simulink model "SOC_Estimation_vk"  (R2018b)
settings: Solver=ode4  StartTime=0.0  StopTime=5000  FixedStep=1e-3  RelTol=1e-3
libraries: nesl_utility x8, fl_lib x7, ee_lib x2
settings Model: Creator=Suresh  LastModifiedBy=Suresh
settings DataIOCC: ReturnWorkspaceOutputs=on

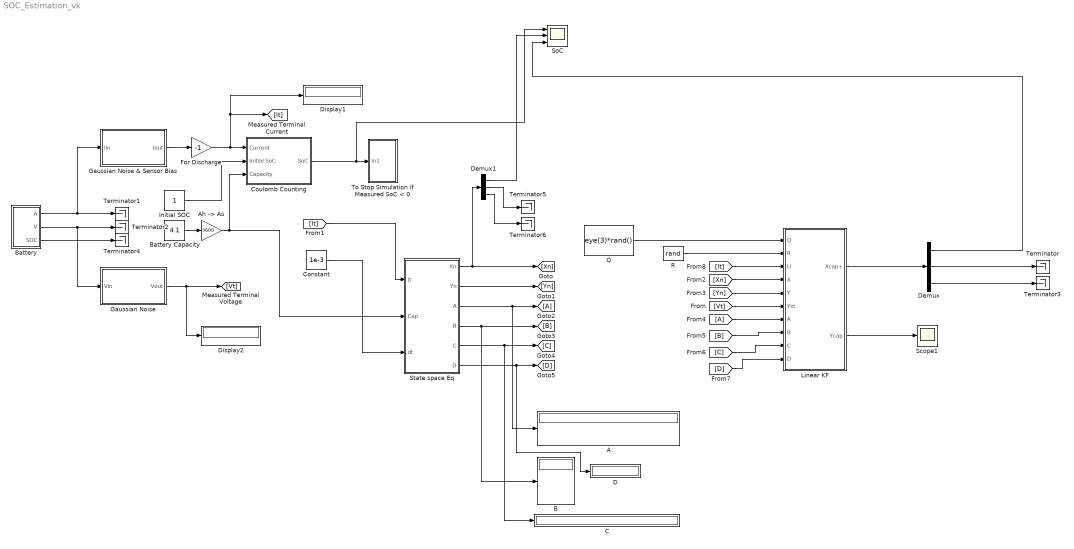
== system SOC_Estimation_vk ==
  A : Display
  "Ah -> As" : Gain  Gain=3600
  B : Display
  Battery : Subsystem
  Battery Capacity : Constant  Value=4.1
  C : Display
  Constant : Constant  Value=1e-3
  "Coulomb Counting " : Subsystem
  D : Display
  Demux : Demux  Outputs=3
  Demux1 : Demux  Outputs=3
  Display1 : Display
  Display2 : Display
  For Discharge : Gain  Gain=-1
  Gaussian Noise : Subsystem
  Gaussian Noise & Sensor Bias : Subsystem
  Initial SOC : Constant
  Linear KF : Subsystem
  Q : Constant  Value=eye(3)*rand()
  R : Constant  Value=rand
  Scope1 : Scope
  SoC : Scope  NumInputPorts=3
  State space Eq : Subsystem
  Terminator{,1..6} (7 alike) : Terminator
  To Stop Simulation if Measured SoC < 0 : Subsystem
  wires:
  Battery/2(V) -> Gaussian Noise/1(Vin), Terminator2/1
  Battery/1(A) -> Gaussian Noise & Sensor Bias/1(Iin), Terminator1/1
  Gaussian Noise & Sensor Bias/1(Iout) -> For Discharge/1
  "Coulomb Counting "/1("SoC ") -> SoC/1, To Stop Simulation if Measured SoC < 0/1(In1)
  Initial SOC/1 -> "Coulomb Counting "/2(Initial SoC)
  Battery/3(SOC) -> Terminator4/1
  Gaussian Noise/1(Vout) -> Display2/1, [Vt]
  Battery Capacity/1 -> "Ah -> As"/1
  For Discharge/1 -> [It], Display1/1, "Coulomb Counting "/1(Current)
  "Ah -> As"/1 -> State space Eq/2(Cap), "Coulomb Counting "/3(Capacity)
  [It] -> State space Eq/1(It)
  Constant/1 -> State space Eq/3(dt)
  State space Eq/1(Xn) -> Demux1/1, [Xn]
  State space Eq/2(Yn) -> [Yn]
  State space Eq/3(A) -> [A], A/1
  State space Eq/4(B) -> [B], B/1
  State space Eq/5(C) -> [C], C/1
  State space Eq/6(D) -> D/1, [D]
  Demux/2 -> Terminator/1
  Demux/3 -> Terminator3/1
  Demux/1 -> SoC/3
  Demux1/1 -> SoC/2
  Demux1/2 -> Terminator5/1
  Demux1/3 -> Terminator6/1
  Q/1 -> Linear KF/1(Q)
  R/1 -> Linear KF/2(R)
  [It] -> Linear KF/3(U)
  [Xn] -> Linear KF/4(X)
  [Yn] -> Linear KF/5(Y)
  [Vt] -> Linear KF/6(Ym)
  [A] -> Linear KF/7(A)
  [B] -> Linear KF/8(B)
  [C] -> Linear KF/9(C)
  [D] -> Linear KF/10(D)
  Linear KF/1(Xcap+) -> Demux/1
  Linear KF/2(Ycap) -> Scope1/1

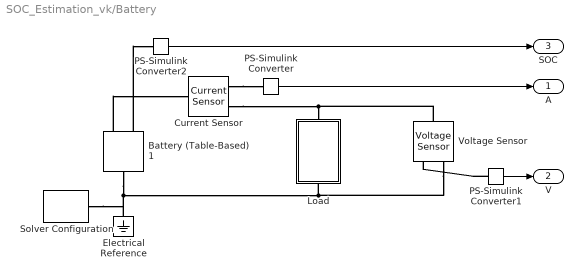
== system SOC_Estimation_vk/Battery ==
  Battery (Table-Based)1 : ee_lib/Sources/Battery (Table-Based)  SOC_vec=[0, .25, .75, 1]  T_vec=[273.15, 298.15, 323.15] K  V0_mat=[3.2, 3.1, 3.14; 3.25, 3.27, 3.3; 3.28, 3.31, 3.34; 3.33, 3.5, 3.59] V  R0_mat=[.03, .015, .002; .04, .017, .008; .039, .012, .006; .027, .013, .021] Ohm  AH_vec=[2.9, 4.1, 4.2] hr*A  prm_leak=1  Rleak_vec=[8000, 7000, 6000] Ohm  prm_dyn=3  R1_mat=[.089, .076, .01; .042, .022, .099; .019, .007, .002; .051, .043, .029] Ohm  tau1_mat=[44, 148, 235; 93, 110, 1000; 19, 27, 133; .5, 22, 3] s  R2_mat=[.014, .382, .407; .028, .006, .007; .014, .007, .006; .333, .956, .912] Ohm  tau2_mat=[1, 44, 5644; 11, 24, 506; 2, 14, 330; 3310, 13419, 30216] s  R3_mat=[.014, .382, .407; .028, .006, .007; .014, .007, .006; .333, .956, .912] Ohm  tau3_mat=[1, 44, 5644; 11, 24, 506; 2, 14, 330; 3310, 13419, 30216] s  R4_mat=[.014, .382, .407; .028, .006, .007; .014, .007, .006; .333, .956, .912] Ohm  tau4_mat=[1, 44, 5644; 11, 24, 506; 2, 14, 330; 3310, 13419, 30216] s  R5_mat=[.014, .382, .407; .028, .006, .007; .014, .007, .006; .333, .956, .912] Ohm  tau5_mat=[1, 44, 5644; 11, 24, 506; 2, 14, 330; 3310, 13419, 30216] s  N0=100  dV0=0  dR0=0  dAH=0  dRleak=0  dR1=0  dR2=0  dR3=0  dR4=0  dR5=0  temperature=298.15 K  i_specify=off  i_priority=None  i=0 A  i_nominal_specify=off  i_nominal_unit=A  i_nominal_value=1  v_specify=off  v_priority=None  v=0 V  v_nominal_specify=off  v_nominal_unit=V  v_nominal_value=1  stateOfCharge_specify=off  stateOfCharge_priority=High  stateOfCharge=1  stateOfCharge_nominal_specify=off  stateOfCharge_nominal_unit=1  stateOfCharge_nominal_value=1  num_cycles_specify=off  num_cycles_priority=High  num_cycles=0  num_cycles_nominal_specify=off  num_cycles_nominal_unit=1  num_cycles_nominal_value=1  thermal_mass=30000 J/K  temperature_specify=off  temperature_priority=High  temperature_nominal_specify=off  temperature_nominal_unit=K  temperature_nominal_value=1
      settings: SourceProductName=Simscape Electrical  SourceProductBaseCode=PS  LogSimulationData=on
  Current Sensor : fl_lib/Electrical/Electrical Sensors/Current Sensor
  Electrical Reference : fl_lib/Electrical/Electrical Elements/Electrical Reference
  Load : Subsystem
  PS-Simulink Converter : nesl_utility/PS-Simulink Converter  PhysicalDomain=network_engine_domain  SubClassName=ps_output  LeftPortType=input  RightPortType=output  PseudoPeriodic=off  Frequencies=[]  Unit=1  AffineConversion=off
  PS-Simulink Converter1 : nesl_utility/PS-Simulink Converter  PhysicalDomain=network_engine_domain  SubClassName=ps_output  LeftPortType=input  RightPortType=output  PseudoPeriodic=off  Frequencies=[]  Unit=1  AffineConversion=off
  PS-Simulink Converter2 : nesl_utility/PS-Simulink Converter  PhysicalDomain=network_engine_domain  SubClassName=ps_output  LeftPortType=input  RightPortType=output  PseudoPeriodic=off  Frequencies=[]  Unit=1  AffineConversion=off
  Solver Configuration : nesl_utility/Solver Configuration  PhysicalDomain=network_engine_domain  SubClassName=solver  LeftPortType=input  RightPortType=generic  Tones=[]  Harmonics=[]  SimulateNoise=off  Profile=off  UseLocalSampling=off  EnableSwitchedLinearOptims=on  FrequencyDomain=off  UseCCode=off  RelTol=0.001  AbsTol=1e-06  MinStep=1e-09  ToWorkspace=off  RevertToSquareIcSolve=off  NumHomotopyIterations=100  PhasorMode=off  PhasorModeNumHarmonics=1  DoDC=off  ResidualTolerance=1e-09  UseLocalSolver=off  LocalSolverChoice=NE_BACKWARD_EULER_ADVANCER  LocalSolverSampleTime=0.001  DoFixedCost=off  MaxNonlinIter=3  MaxModeIter=2  LinearAlgebra=auto  EquationFormulation=NE_TIME_EF  DelaysMemoryBudget=1024  AutomaticFiltering=on  FilteringTimeConstant=0.001  PartitionStorageMethod=AS_NEEDED  PartitionMemoryBudget=1024  PartitionMethod=ROBUST
  Voltage Sensor : fl_lib/Electrical/Electrical Sensors/Voltage Sensor
  A : Outport
  V : Outport  Port=2
  SOC : Outport  Port=3
  wires:
  PS-Simulink Converter/1 -> A/1
  PS-Simulink Converter1/1 -> V/1
  PS-Simulink Converter2/1 -> SOC/1
  connections:
  PS-Simulink Converter1/LConn1 -- Voltage Sensor/RConn1
  Current Sensor/RConn2 -- Voltage Sensor/LConn1 -- Load/LConn1
  Battery (Table-Based)1/LConn1 -- Current Sensor/LConn1
  Current Sensor/RConn1 -- PS-Simulink Converter/LConn1
  Battery (Table-Based)1/LConn2 -- PS-Simulink Converter2/LConn1
  Voltage Sensor/RConn2 -- Load/RConn1 -- Battery (Table-Based)1/RConn1 -- Solver Configuration/RConn1 -- Electrical Reference/LConn1

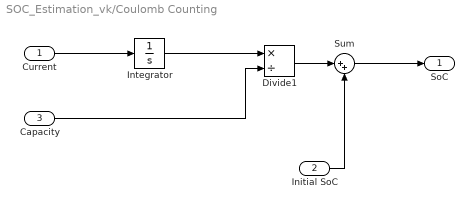
== system SOC_Estimation_vk/Coulomb Counting  ==
  Current : Inport
  Initial SoC : Inport  Port=2
  Capacity : Inport  Port=3
  Divide1 : Product  Inputs=*/
  Integrator : Integrator  LimitOutput=on
  Sum : Sum  Inputs=|++
  "SoC " : Outport
  wires:
  Current/1 -> Integrator/1
  Integrator/1 -> Divide1/1
  Divide1/1 -> Sum/1
  Sum/1 -> "SoC "/1
  Initial SoC/1 -> Sum/2
  Capacity/1 -> Divide1/2

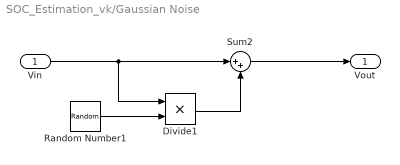
== system SOC_Estimation_vk/Gaussian Noise ==
  Vin : Inport
  Divide1 : Product
  Random Number1 : RandomNumber  Variance=0.000025  Seed=100  SampleTime=1
  Sum2 : Sum  Inputs=|++
  Vout : Outport
  wires:
  Sum2/1 -> Vout/1
  Random Number1/1 -> Divide1/2
  Vin/1 -> Sum2/1, Divide1/1
  Divide1/1 -> Sum2/2

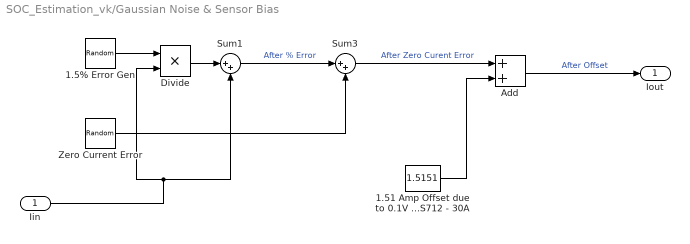
== system SOC_Estimation_vk/Gaussian Noise & Sensor Bias ==
  Iin : Inport
  1.5% Error Gen : RandomNumber  Variance=0.000025  Seed=101  SampleTime=1
  1.51 Amp Offset due to 0.1V Bias measured from Current Sensor ACS712 - 30A : Constant  Value=1.5151
  Add : Sum
  Divide : Product
  Sum1 : Sum  Inputs=|++
  Sum3 : Sum  Inputs=|++
  Zero Current Error : RandomNumber  Variance=0.0003124  Seed=101  SampleTime=1
  Iout : Outport
  wires:
  Iin/1 -> Sum1/2, Divide/2
  Sum1/1 -> Sum3/1  "After % Error"
  Divide/1 -> Sum1/1
  Sum3/1 -> Add/1  "After Zero Curent Error"
  Zero Current Error/1 -> Sum3/2
  1.5% Error Gen/1 -> Divide/1
  1.51 Amp Offset due to 0.1V Bias measured from Current Sensor ACS712 - 30A/1 -> Add/2
  Add/1 -> Iout/1  "After Offset"

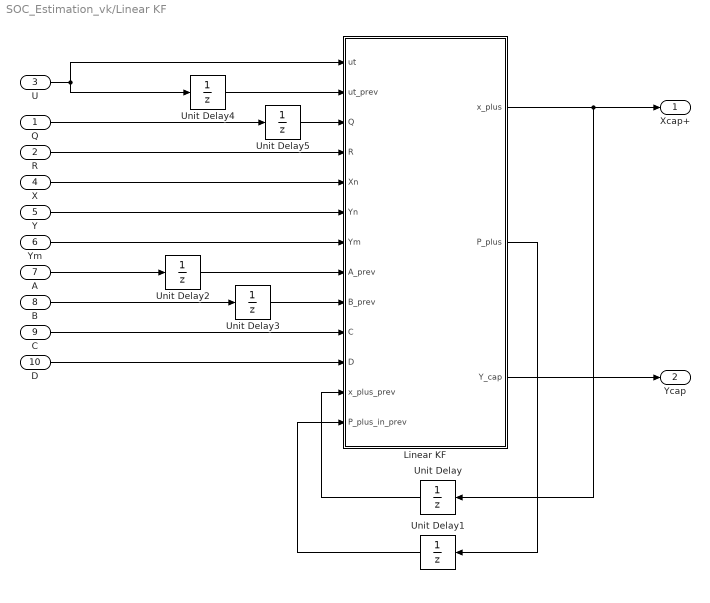
== system SOC_Estimation_vk/Linear KF ==
  Q : Inport
  R : Inport  Port=2
  U : Inport  Port=3
  X : Inport  Port=4
  Y : Inport  Port=5
  Ym : Inport  Port=6
  A : Inport  Port=7
  B : Inport  Port=8
  C : Inport  Port=9
  D : Inport  Port=10
  Linear KF : MATLAB Function  TreatAsAtomicUnit=on
  Unit Delay : UnitDelay  InitialCondition=[1;0;0]  SampleTime=-1  HasFrameUpgradeWarning=on
  Unit Delay1 : UnitDelay  InitialCondition=zeros(3)  SampleTime=-1  HasFrameUpgradeWarning=on
  Unit Delay2 : UnitDelay  InitialCondition=eye(3)  SampleTime=-1  HasFrameUpgradeWarning=on
  Unit Delay3 : UnitDelay  InitialCondition=[0; 0; 0]  SampleTime=-1  HasFrameUpgradeWarning=on
  Unit Delay4 : UnitDelay  SampleTime=-1  HasFrameUpgradeWarning=on
  Unit Delay5 : UnitDelay  InitialCondition=zeros(3)  SampleTime=-1  HasFrameUpgradeWarning=on
  Xcap+ : Outport
  Ycap : Outport  Port=2
  wires:
  Unit Delay2/1 -> Linear KF/8(A_prev)
  U/1 -> Unit Delay4/1, Linear KF/1(ut)
  Unit Delay/1 -> Linear KF/12(x_plus_prev)
  Unit Delay3/1 -> Linear KF/9(B_prev)
  Linear KF/2(P_plus) -> Unit Delay1/1
  Unit Delay1/1 -> Linear KF/13(P_plus_in_prev)
  Unit Delay5/1 -> Linear KF/3(Q)
  B/1 -> Unit Delay3/1
  Linear KF/1(x_plus) -> Unit Delay/1, Xcap+/1
  Unit Delay4/1 -> Linear KF/2(ut_prev)
  Q/1 -> Unit Delay5/1
  A/1 -> Unit Delay2/1
  C/1 -> Linear KF/10(C)
  D/1 -> Linear KF/11(D)
  Linear KF/3(Y_cap) -> Ycap/1
  R/1 -> Linear KF/4(R)
  Y/1 -> Linear KF/6(Yn)
  Ym/1 -> Linear KF/7(Ym)
  X/1 -> Linear KF/5(Xn)

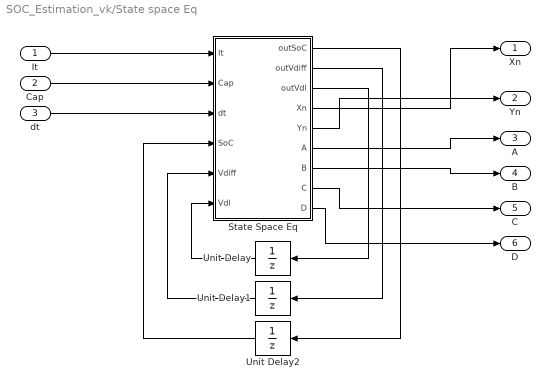
== system SOC_Estimation_vk/State space Eq ==
  It : Inport
  Cap : Inport  Port=2
  dt : Inport  Port=3
  State Space Eq : MATLAB Function  TreatAsAtomicUnit=on
  Unit Delay : UnitDelay  SampleTime=-1  HasFrameUpgradeWarning=on
  Unit Delay1 : UnitDelay  SampleTime=-1  HasFrameUpgradeWarning=on
  Unit Delay2 : UnitDelay  InitialCondition=1  SampleTime=-1  HasFrameUpgradeWarning=on
  Xn : Outport
  Yn : Outport  Port=2
  A : Outport  Port=3
  B : Outport  Port=4
  C : Outport  Port=5
  D : Outport  Port=6
  wires:
  State Space Eq/6(A) -> A/1
  State Space Eq/9(D) -> D/1
  State Space Eq/2(outVdiff) -> Unit Delay1/1
  Unit Delay2/1 -> State Space Eq/4(SoC)
  State Space Eq/1(outSoC) -> Unit Delay2/1
  Unit Delay1/1 -> State Space Eq/5(Vdiff)
  State Space Eq/3(outVdl) -> Unit Delay/1
  State Space Eq/8(C) -> C/1
  Unit Delay/1 -> State Space Eq/6(Vdl)
  It/1 -> State Space Eq/1(It)
  dt/1 -> State Space Eq/3(dt)
  Cap/1 -> State Space Eq/2(Cap)
  State Space Eq/7(B) -> B/1
  State Space Eq/4(Xn) -> Xn/1
  State Space Eq/5(Yn) -> Yn/1

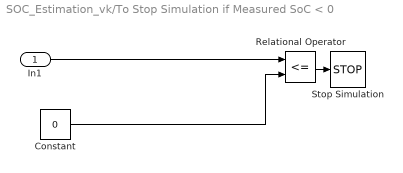
== system SOC_Estimation_vk/To Stop Simulation if Measured SoC < 0 ==
  In1 : Inport
  Constant : Constant  Value=0
  Relational Operator : RelationalOperator  Operator=<=  OutDataTypeStr=boolean  RndMeth=Simplest
  Stop Simulation : Stop
  wires:
  Relational Operator/1 -> Stop Simulation/1
  Constant/1 -> Relational Operator/2
  In1/1 -> Relational Operator/1

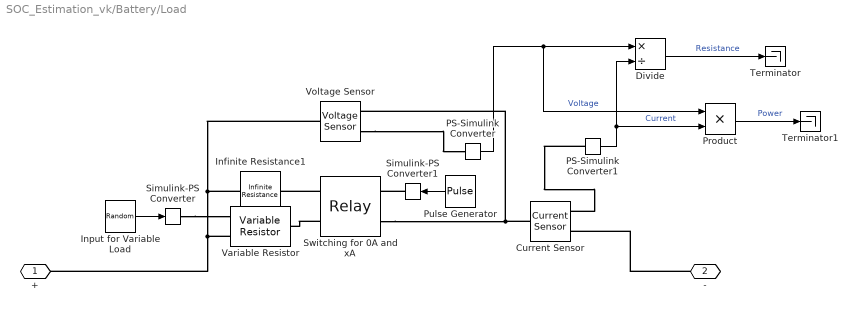
== system SOC_Estimation_vk/Battery/Load ==
  Current Sensor : fl_lib/Electrical/Electrical Sensors/Current Sensor
  Divide : Product  Inputs=*/
  Infinite Resistance1 : fl_lib/Electrical/Electrical Elements/Infinite Resistance  v_specify=off  v_priority=None  v=0 V  v_nominal_specify=off  v_nominal_unit=V  v_nominal_value=1
      settings: SourceProductName=Simscape  SourceProductBaseCode=SS
  Input for Variable Load : UniformRandomNumber  Minimum=0.01  Maximum=1.0  Seed=100  SampleTime=200
  PS-Simulink Converter : nesl_utility/PS-Simulink Converter  PhysicalDomain=network_engine_domain  SubClassName=ps_output  LeftPortType=input  RightPortType=output  PseudoPeriodic=off  Frequencies=[]  Unit=1  AffineConversion=off
  PS-Simulink Converter1 : nesl_utility/PS-Simulink Converter  PhysicalDomain=network_engine_domain  SubClassName=ps_output  LeftPortType=input  RightPortType=output  PseudoPeriodic=off  Frequencies=[]  Unit=1  AffineConversion=off
  Product : Product
  Pulse Generator : DiscretePulseGenerator  PulseType=Time based  Period=500  PulseWidth=40
  Simulink-PS Converter : nesl_utility/Simulink-PS Converter  PhysicalDomain=network_engine_domain  SubClassName=ps_input  LeftPortType=input  RightPortType=output  PseudoPeriodic=off  Frequencies=[]  NoiseDistribution=none  NoiseParameters=[]  Unit=1  AffineConversion=off  FilteringAndDerivatives=zero  SimscapeFilterOrder=1  InputFilterTimeConstant=0.001  UdotUserProvided=0
  Simulink-PS Converter1 : nesl_utility/Simulink-PS Converter  PhysicalDomain=network_engine_domain  SubClassName=ps_input  LeftPortType=input  RightPortType=output  PseudoPeriodic=off  Frequencies=[]  NoiseDistribution=none  NoiseParameters=[]  Unit=1  AffineConversion=off  FilteringAndDerivatives=provide  SimscapeFilterOrder=1  InputFilterTimeConstant=0.001  UdotUserProvided=0
  Switching for 0A and xA : ee_lib/Switches & Breakers/Relay  T_brk_C_S1=0 s  T_mak_C_S1=0 s  T_brk_C_S2=0 s  T_mak_C_S2=0 s  R_closed=0.01 Ohm  G_open=1e-8 1/Ohm  Threshold=0.9  exposemeasurement=ee.enum.exposemeasurement.hidden
      settings: SourceProductName=Simscape Electrical  SourceProductBaseCode=PS
  Terminator : Terminator
  Terminator1 : Terminator
  Variable Resistor : fl_lib/Electrical/Electrical Elements/Variable Resistor  Rmin=0 Ohm  i_specify=off  i_priority=None  i=0 A  i_nominal_specify=off  i_nominal_unit=A  i_nominal_value=1  v_specify=off  v_priority=None  v=0 V  v_nominal_specify=off  v_nominal_unit=V  v_nominal_value=1
  Voltage Sensor : fl_lib/Electrical/Electrical Sensors/Voltage Sensor
  + : PMIOPort  Side=Left
  - : PMIOPort  Port=2  Side=Right
  wires:
  PS-Simulink Converter/1 -> Product/1, Divide/1  "Voltage"
  PS-Simulink Converter1/1 -> Product/2, Divide/2  "Current"
  Divide/1 -> Terminator/1  "Resistance"
  Product/1 -> Terminator1/1  "Power"
  Pulse Generator/1 -> Simulink-PS Converter1/1
  Input for Variable Load/1 -> Simulink-PS Converter/1
  connections:
  Voltage Sensor/LConn1 -- Infinite Resistance1/LConn1 -- Variable Resistor/LConn2 -- +/RConn1
  Current Sensor/LConn1 -- Switching for 0A and xA/LConn2 -- Voltage Sensor/RConn2
  -/RConn1 -- Current Sensor/RConn2
  Voltage Sensor/RConn1 -- PS-Simulink Converter/LConn1
  PS-Simulink Converter1/LConn1 -- Current Sensor/RConn1
  Switching for 0A and xA/RConn1 -- Infinite Resistance1/RConn1
  Switching for 0A and xA/RConn2 -- Variable Resistor/RConn1
  Simulink-PS Converter/RConn1 -- Variable Resistor/LConn1
  Simulink-PS Converter1/RConn1 -- Switching for 0A and xA/LConn1

== matlab function SOC_Estimation_vk/Linear KF/Linear KF ==
  data: ut input; ut_prev input; Q input; x_plus output; R input; Xn input; Yn input; Ym input; A_prev input; B_prev input; P_plus output; C input; D input; x_plus_prev input; P_plus_in_prev input; Y_cap output
function [x_plus,P_plus,Y_cap] = fcn(ut,ut_prev,Q,R,Xn,Yn,Ym,A_prev,B_prev,C,D,x_plus_prev,P_plus_in_prev)

P_minus = A_prev * P_plus_in_prev * A_prev'  + Q;

K = (P_minus * C') /(C * P_minus * C' + R);

x_minus = A_prev * x_plus_prev + B_prev * ut_prev; 

x_plus = x_minus + K * (Ym - C * x_minus);

P_plus = (eye(length(K*C)) - K*C)*P_minus;

Y_cap = C*x_plus + D*ut; %output eq with xcap


end

== matlab function SOC_Estimation_vk/State space Eq/State Space Eq ==
  data: outSoC output; It input; Cap input; dt input; outVdiff output; outVdl output; SoC input; Vdiff input; Vdl input; Xn output; Yn output; A output; B output; C output; D output
function [outSoC,outVdiff,outVdl,Xn,Yn,A,B,C,D] = fcn(It,Cap,dt,SoC,Vdiff,Vdl)

Rohm = @(SoC) 0.04267*(SoC).^3 - 0.06667*(SoC).^2 + 0.022 * (SoC) + 0.015;
Rdiff = @(SoC) 0.006326*exp((-2.269)*SoC) + 0.0006345*exp(3.837*SoC);
Cdiff = @(SoC) 4533*(SoC).^3 - 23860*(SoC).^2 + 17890*(SoC) + 1947; 
Rdl = @(SoC) (9.469e-05)*exp((-7.579*SoC)) + (5.1810e-05)*exp(8.967*SoC);
Cdl = @(SoC) 95580*(SoC).^3 - 121600*(SoC).^2 + 39970*(SoC) + 115.2; 
Voc = @(SoC) 1.707*(SoC).^3 - 2.507*(SoC).^2 + 1.2 *(SoC)+ 3.1;
VocPrime = @(SoC) (5121*(SoC.^2))/1000 - (2507*SoC)/500 + 6/5; %derivative

tau1 = @(SoC) 0.2133*(SoC^3) - 0.232*(SoC^2) - 0.1073*(SoC) + 0.148;
tau2 = @(SoC) 44*exp(-2.425*SoC) + (9.17e-10)*exp(30.31*SoC);

X = [SoC;
    Vdiff;
    Vdl];

A = [1, 0, 0;
    0, 1-(dt/tau1(X(1))),0;
    0,0,1-(dt/tau2(X(1)))];

B = [dt/Cap;
    dt/(tau1(X(1))/Rdiff(X(1)));
    dt/(tau2(X(1))/Rdl(X(1)))];

C = [VocPrime(X(1)), 1, 1];
    
D = Rohm(X(1));

Xn = A*X + B*It;
Yn = C*X + D*It;

% if(time==0)
%     outSoC = 1;
%     outVdiff = 0;
%     outVdl = 0;
% else
    outSoC = Xn(1);
    outVdiff = Xn(2);
    outVdl = Xn(3);
% end

end
